simulink model "PIDTuningNoControl"  (R2017a)
settings: Solver=VariableStepAuto  StartTime=0.0  StopTime=duur  RelTol=1e-3  EnableMultiTasking=on
values from neighbouring files (symbols this model uses):
  K = sys.num/sys.den(2)    [PIDTuning.m]
  tau = 1/sys.den(2)    [PIDTuning.m]    (also in controlWithMeasurementDelay.m = 300; margin.m = 300)
  td = 1.5    [PIDTuning.m]    (also in controlWithMeasurementDelay.m = 120)
settings Model: Creator=wrquaghe  LastModifiedBy=geert
settings DataIOCC: LimitDataPoints=on
settings OptimizationCC: LifeSpan=inf
settings DebuggingCC: AllowSymbolicDim=off  SFUnexpectedBacktrackingDiag=warning  SFNoUnconditionalDefaultTransitionDiag=warning  SFExecutionAtInitializationDiag=none
settings ModelReferenceCC: PropagateSignalLabelsOutOfModel=off
settings GRTTargetCC: TargetLangStandard=C89/C90 (ANSI)
settings ConfigComp: CovMetricSettings=dw  CovHtmlReporting=on  CovSaveCumulativeToWorkspaceVar=on  CovSaveSingleToWorkspaceVar=on  CovExternalEMLEnable=off

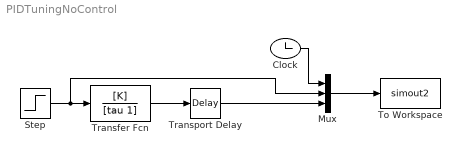
== system PIDTuningNoControl ==
  Clock : Clock
  Mux : Mux  Inputs=3
  Step : Step  SampleTime=0
  To Workspace : ToWorkspace  VariableName=simout2  SampleTime=1
  Transfer Fcn : TransferFcn  Numerator=[K]  Denominator=[tau 1]
  Transport Delay : TransportDelay  DelayTime=td
  wires:
  Step/1 -> Mux/2, Transfer Fcn/1
  Clock/1 -> Mux/1
  Mux/1 -> To Workspace/1
  Transfer Fcn/1 -> Transport Delay/1
  Transport Delay/1 -> Mux/3
